simulink model "rtwdemo_typeconvsf"  (Simulink 7.1)
settings: Solver=FixedStepDiscrete  StartTime=0.0  StopTime=10.0  RelTol=1e-3
settings Model: Creator=ajayaram  LastModifiedBy=ajayaram
settings OptimizationCC: InlineParams=on  OptimizeModelRefInitCode=on  LifeSpan=1
settings RTWCC: SystemTargetFile=ert.tlc  GenCodeOnly=on  GenerateMakefile=off  TemplateMakefile=ert_default_tmf  Description=Real-Time Workshop Embedded Coder (no auto configuration)  GenerateReport=on  ProcessScript=ert_make_rtw_hook  IncludeHyperlinkInReport=on  LaunchReport=on
settings CodeAppCC: GenerateComments=off  IgnoreCustomStorageClasses=off  SimulinkBlockComments=off
settings ERTTargetCC: GenerateSampleERTMain=on  InlinedParameterPlacement=NonHierarchical  ERTCustomFileTemplate=example_file_process.tlc

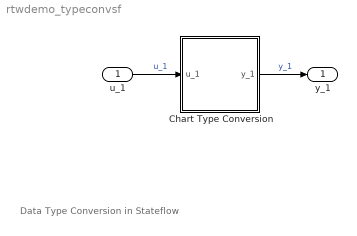
== system rtwdemo_typeconvsf ==
  note: Data Type Conversion in Stateflow
  u_1 : Inport  DataType=int32  OutDataType=sfix(16)  OutScaling=2^0  OutDataTypeStr=int32
  Chart Type Conversion : Stateflow chart
  y_1 : Outport  OutDataType=sfix(16)  OutScaling=2^0
  wires:
  u_1/1 -> Chart Type Conversion/1(u_1)  "u_1"
  Chart Type Conversion/1(y_1) -> y_1/1  "y_1"

== stateflow chart Chart Type Conversion ==
  (default) -> (junction 3)
  (junction 3) -> (junction 4) : {
      | y_1= double ( u_1 );
      | }
  data: u_1 input double; y_1 output single
